simulink model "harmonic_analysis"  (R2016a)
settings: Solver=VariableStepAuto  StartTime=0.0  StopTime=Tfinal1  RelTol=1e-3
values from neighbouring files (symbols this model uses):
  Ts1 = 0.1e-6    (= 1e-07)    [cizdir.m]
libraries: powerlib_meascontrol x9, powerlib x1
settings Model: Creator=mesutto  LastModifiedBy=mesutto

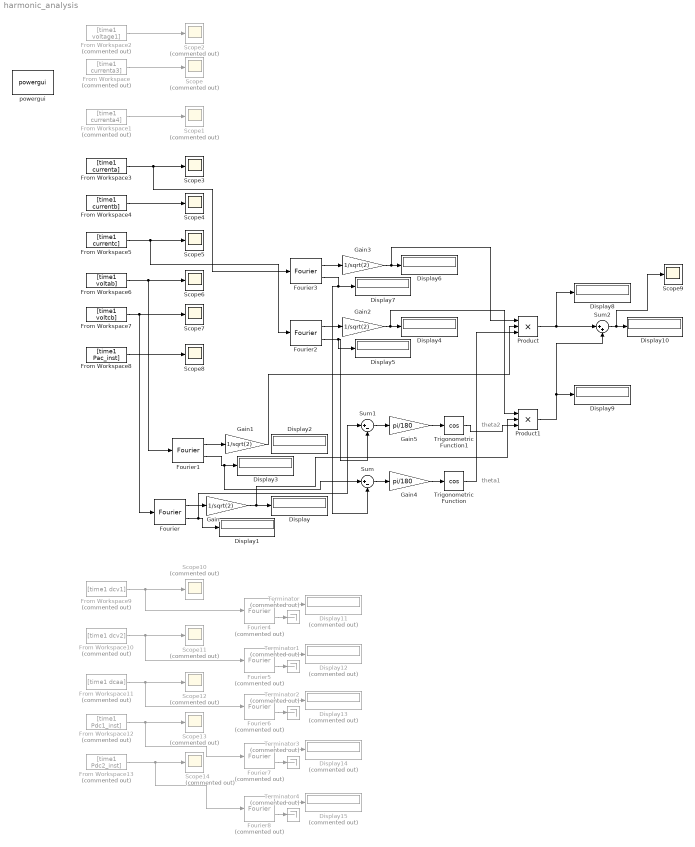
== system harmonic_analysis ==
  note: theta1
  note: theta2
  Display{,1..10} (11 alike) : Display
  Display{11..15} (5 alike) : Display  Commented=on
  Fourier{,1..3} (4 alike) : powerlib_meascontrol/Measurements/Fourier  Freq=50  n=1  InInit=[0, 0]  Ts=0
  Fourier{4..8} (5 alike) : powerlib_meascontrol/Measurements/Fourier  Commented=on  Freq=50  n=0  InInit=[0, 0]  Ts=0
  From Workspace : FromWorkspace  Commented=on  VariableName=[time1 currenta3]  OutDataTypeStr=double  SampleTime=Ts1
  From Workspace1 : FromWorkspace  Commented=on  VariableName=[time1 currenta4]  OutDataTypeStr=double  SampleTime=Ts1
  From Workspace10 : FromWorkspace  Commented=on  VariableName=[time1 dcv2]  OutDataTypeStr=double  SampleTime=Ts1
  From Workspace11 : FromWorkspace  Commented=on  VariableName=[time1 dcaa]  OutDataTypeStr=double  SampleTime=Ts1
  From Workspace12 : FromWorkspace  Commented=on  VariableName=[time1 Pdc1_inst]  OutDataTypeStr=double  SampleTime=Ts1
  From Workspace13 : FromWorkspace  Commented=on  VariableName=[time1 Pdc2_inst]  OutDataTypeStr=double  SampleTime=Ts1
  From Workspace2 : FromWorkspace  Commented=on  VariableName=[time1 voltage1]  OutDataTypeStr=double  SampleTime=Ts1
  From Workspace3 : FromWorkspace  VariableName=[time1 currenta]  OutDataTypeStr=double  SampleTime=Ts1
  From Workspace4 : FromWorkspace  VariableName=[time1 currentb]  OutDataTypeStr=double  SampleTime=Ts1
  From Workspace5 : FromWorkspace  VariableName=[time1 currentc]  OutDataTypeStr=double  SampleTime=Ts1
  From Workspace6 : FromWorkspace  VariableName=[time1 voltab]  OutDataTypeStr=double  SampleTime=Ts1
  From Workspace7 : FromWorkspace  VariableName=[time1 voltcb]  OutDataTypeStr=double  SampleTime=Ts1
  From Workspace8 : FromWorkspace  VariableName=[time1 Pac_inst]  OutDataTypeStr=double  SampleTime=Ts1
  From Workspace9 : FromWorkspace  Commented=on  VariableName=[time1 dcv1]  OutDataTypeStr=double  SampleTime=Ts1
  Gain{,1..3} (4 alike) : Gain  Gain=1/sqrt(2)
  Gain4 : Gain  Gain=pi/180
  Gain5 : Gain  Gain=pi/180
  Product : Product  Inputs=3
  Product1 : Product  Inputs=3
  Scope{,1..2,10..14} (8 alike) : Scope  Commented=on
  Scope{3..9} (7 alike) : Scope
  Sum : Sum  Inputs=|+-
  Sum1 : Sum  Inputs=|+-
  Sum2 : Sum  Inputs=|++
  Terminator{,1..4} (5 alike) : Terminator  Commented=on
  Trigonometric Function : Trigonometry  Operator=cos
  Trigonometric Function1 : Trigonometry  Operator=cos
  powergui : powerlib/powergui  Priority=1  SimulationMode=Discrete  SolverType=Tustin/Backward Euler (TBE)  SampleTime=Ts1  frequency=60  SPID=off  DisableSnubberDevices=off  DisableRonSwitches=off  DisableVfSwitches=off  SwTol=0  DisplayEquations=off  Interpol=off  ExternalGateDelay=off  methode=off  Ts=10  FunctionMessages=off  echomessages=off  HookPort=off  EnableUseOfTLC=off  x0status=blocks  frequencyindice=60  Pbase=100e6  ErrMax=1e-4  Iterations=50  UnitsV=kV  UnitsW=MW  buscounter=0  RestoreLinks=warning  ResistiveCurrentMeasurement=off  Frange=[0:2:500]  Ylog=off  Xlog=on  ShowGrid=off  save=off  variable=ZData  structure=Pdc2  ZoomFFT=off  StartTime=0  cycles=2  DisplayStyle=5  fundamental=50  FreqAxis=off  MaxFrequency=200000  frequencyindicesteady=1  RmsSteady=1  display=off
  wires:
  From Workspace/1 -> Scope/1
  From Workspace1/1 -> Scope1/1
  From Workspace2/1 -> Scope2/1
  From Workspace3/1 -> Fourier3/1, Scope3/1
  From Workspace4/1 -> Scope4/1
  From Workspace5/1 -> Fourier2/1, Scope5/1
  From Workspace6/1 -> Fourier1/1, Scope6/1
  From Workspace7/1 -> Fourier/1, Scope7/1
  From Workspace8/1 -> Scope8/1
  Fourier/1 -> Gain/1
  Fourier/2 -> Sum1/1, Display1/1
  Gain/1 -> Product1/2, Display/1
  Fourier1/1 -> Gain1/1
  Fourier1/2 -> Sum/1, Display3/1
  Gain1/1 -> Product/2
  Fourier2/1 -> Gain2/1
  Fourier2/2 -> Sum1/2, Display5/1
  Fourier3/1 -> Gain3/1
  Fourier3/2 -> Display7/1, Sum/2
  Sum/1 -> Gain4/1
  Gain4/1 -> Trigonometric Function/1
  Gain5/1 -> Trigonometric Function1/1
  Sum1/1 -> Gain5/1
  Trigonometric Function/1 -> Product/3
  Gain3/1 -> Product/1, Display6/1
  Gain2/1 -> Product1/1, Display4/1
  Trigonometric Function1/1 -> Product1/3
  Product/1 -> Sum2/1, Display8/1
  Product1/1 -> Sum2/2, Display9/1
  Sum2/1 -> Scope9/1, Display10/1
  From Workspace9/1 -> Fourier4/1, Scope10/1
  Fourier4/1 -> Display11/1
  Fourier4/2 -> Terminator/1
  From Workspace10/1 -> Fourier5/1, Scope11/1
  Fourier5/1 -> Display12/1
  Fourier5/2 -> Terminator1/1
  From Workspace11/1 -> Fourier6/1, Scope12/1
  Fourier6/1 -> Display13/1
  Fourier6/2 -> Terminator2/1
  From Workspace12/1 -> Fourier7/1, Scope13/1
  Fourier7/1 -> Display14/1
  Fourier7/2 -> Terminator3/1
  From Workspace13/1 -> Fourier8/1, Scope14/1
  Fourier8/1 -> Display15/1
  Fourier8/2 -> Terminator4/1
